simulink library "INT_FlFWLvl_VD"  (R2016b)
settings: Solver=VariableStepAuto  StartTime=0.0  StopTime=10.0  RelTol=1e-3
settings Model: Creator=胡炎林  LastModifiedBy=胡炎林

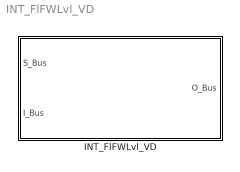
== system INT_FlFWLvl_VD ==
  INT_FlFWLvl_VD : Subsystem

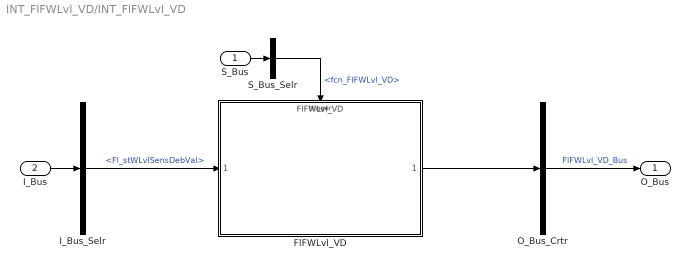
== system INT_FlFWLvl_VD/INT_FlFWLvl_VD ==
  S_Bus : Inport
  I_Bus : Inport  Port=2
  FlFWLvl_VD : ModelReference  ModelNameDialog=FlFWLvl_VD  SimulationMode=Normal  ModelReferenceVersion=1.5  TriggerPortName=function  TriggerPortTriggerType=function-call  TriggerPortStatesWhenEnabling=held
  I_Bus_Selr : BusSelector  OutputSignals=Fl_stWLvlSensDebVal
  O_Bus_Crtr : BusCreator  Inputs=1
  S_Bus_Selr : BusSelector  OutputSignals=fcn_FlFWLvl_VD
  O_Bus : Outport
  wires:
  S_Bus_Selr/1 -> FlFWLvl_VD/Trigger  "<fcn_FlFWLvl_VD>"
  S_Bus/1 -> S_Bus_Selr/1
  I_Bus/1 -> I_Bus_Selr/1
  I_Bus_Selr/1 -> FlFWLvl_VD/1  "<Fl_stWLvlSensDebVal>"
  O_Bus_Crtr/1 -> O_Bus/1  "FlFWLvl_VD_Bus"
  FlFWLvl_VD/1 -> O_Bus_Crtr/1
